simulink model "rc_second_order_open_close_loop_P_PI_PID_arduino"  (R2022b)
settings: Solver=FixedStepDiscrete  StartTime=0.0  StopTime=60.0  FixedStep=1e-3  RelTol=1e-3  EnableMultiTasking=on
undefined symbols (not defined in the file): DiscIntNeverNeededParam
libraries: arduinolib x10, simulink x1
settings Model: ExtModeTrigDuration=2  Creator=yasso  LastModifiedBy=yasso
settings OptimizationCC: EnhancedBackFolding=on  PassReuseOutputArgsAs=Individual arguments  ZeroExternalMemoryAtStartup=off  ZeroInternalMemoryAtStartup=off  MaxStackSize=64  OptimizeBlockOrder=speed  DifferentSizesBufferReuse=on  OptimizationCustomize=off  EfficientTunableParamExpr=on
settings DebuggingCC: ParameterTunabilityLossMsg=error
settings HardwareCC: ProdBitPerInt=16  ProdBitPerPointer=16  ProdBitPerSizeT=16  ProdBitPerPtrDiffT=16  ProdLargestAtomicFloat=None  ProdWordSize=8  ProdHWDeviceType=Atmel->AVR
settings SFSimCC: MATLABDynamicMemAlloc=off
settings RTWCC: Description=Embedded Coder  SystemTargetFile=ert.tlc  HardwareBoard=Arduino Uno  TLCOptions=-aInlineSetEventsForThisBaseRateFcn=TLC_FALSE -aSuppressMultiTaskScheduler=TLC_FALSE -aRateBasedStepFcn=1  TemplateMakefile=ert_default_tmf  Toolchain=Arduino AVR  BuildConfiguration=Faster Runs
settings CodeAppCC: ForceParamTrailComments=on  IgnoreCustomStorageClasses=off  OperatorAnnotations=on  SimulinkDataObjDesc=on  SFDataObjDesc=on  InsertBlockDesc=on
settings ERTTargetCC: SupportContinuousTime=on  SupportVariableSizeSignals=on  ExtModeTransport=3  ExtModeStaticAlloc=on  ExtModeAutomaticAllocSize=off  ExtModeStaticAllocSize=250  ExtModeMexFile=ext_xcp  ExtModeIntrfLevel=Level2 - Open

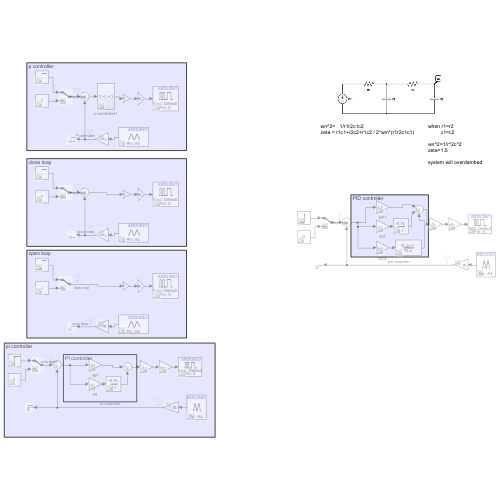
[thumbnail: Simulink's stored preview of the top-level diagram]
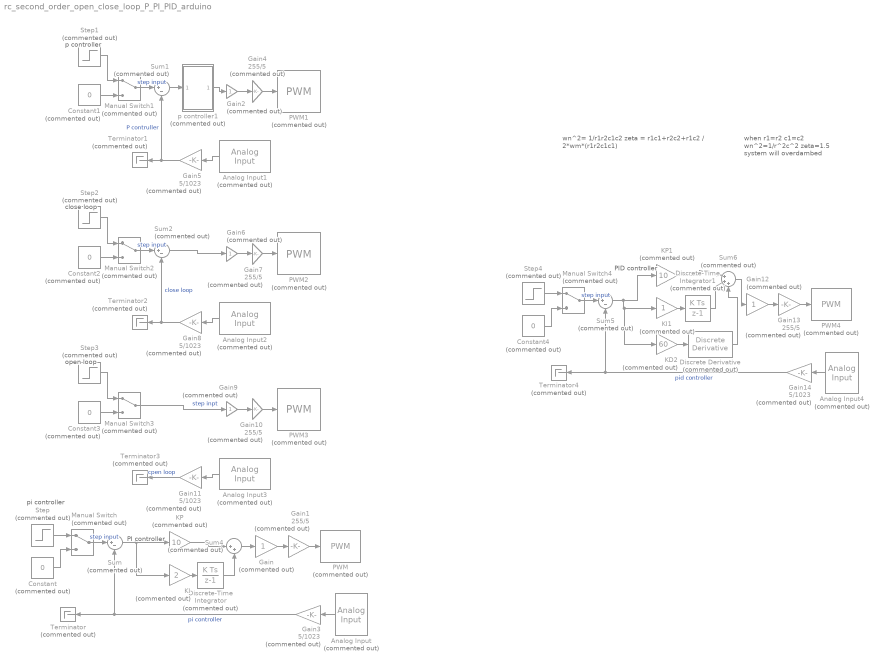
== system rc_second_order_open_close_loop_P_PI_PID_arduino ==
  note: pi controller
  note: PI controller
  note: p controller
  note: when r1=r2
      | c1=c2
      |
      | wn^2=1/r^2c^2
      | zeta=1.5
      |
      | system will overdambed
  note: wn^2= 1/r1r2c1c2
      | zeta = r1c1+r2c2+r1c2 / 2*wm*(r1r2c1c1)
  note: close loop
  note: open loop
  note: PID controller
  Analog Input{,1..4} (5 alike) : arduinolib/Analog Input  Commented=on  pinNumber=4  ReadResultsOnly=off  ConversionTriggerSource=Software  ExternalTriggerType=uint32( 0 )  OutputDataType=uint16  EnableConversionCompleteNotify=off  EnableOuputStatus=off  SampleTime=-1  blockPlatform=arduino
  Constant{,1..4} (5 alike) : Constant  Commented=on  Value=0
  Discrete Derivative : simulink/Discrete/Discrete Derivative  Commented=on  gainval=1.0  ICPrevScaledInput=0.0  OutMin=[]  OutMax=[]  OutDataType=fixdt(1, 16)  OutScaling=2^-10  DoSatur=off
  Discrete-Time Integrator : DiscreteIntegrator  Commented=on  SampleTime=-1  ICPrevOutput=DiscIntNeverNeededParam  ICPrevScaledInput=DiscIntNeverNeededParam
  Discrete-Time Integrator1 : DiscreteIntegrator  Commented=on  SampleTime=-1  ICPrevOutput=DiscIntNeverNeededParam  ICPrevScaledInput=DiscIntNeverNeededParam
  Gain{,2,6,9,12} (5 alike) : Gain  Commented=on
  Gain{1,4,7,10,13} (5 alike) : Gain  Commented=on  Gain=255/5
  Gain{3,5,8,11,14} (5 alike) : Gain  Commented=on  Gain=5/1023
  KD2 : Gain  Commented=on  Gain=60
  KI : Gain  Commented=on  Gain=2
  KI1 : Gain  Commented=on
  KP : Gain  Commented=on  Gain=10
  KP1 : Gain  Commented=on  Gain=10
  Manual Switch{,1..4} (5 alike) : ManualSwitch  Commented=on
  PWM{,1..4} (5 alike) : arduinolib/PWM  Commented=on  pinNumber=5  frequencyType=Default  desiredFrequency=490.2  achievableFrequency=490.2
  Step{,1..4} (5 alike) : Step  Commented=on  SampleTime=0
  Sum{,1..2,5} (4 alike) : Sum  Commented=on  Inputs=|+-
  Sum4 : Sum  Commented=on  Inputs=|++
  Sum6 : Sum  Commented=on  Inputs=|+++
  Terminator{,1..4} (5 alike) : Terminator  Commented=on
  p controller1 : Subsystem  Commented=on
  wires:
  Constant/1 -> Manual Switch/2
  Step/1 -> Manual Switch/1
  Gain/1 -> Gain1/1
  Gain1/1 -> PWM/1
  Analog Input/1 -> Gain3/1
  Gain3/1 -> Sum/2, Terminator/1  "pi controller"
  Manual Switch/1 -> Sum/1  "step input"
  Sum4/1 -> Gain/1
  p controller1/1(Out1) -> Gain2/1
  Sum1/1 -> p controller1/1(In1)
  Manual Switch1/1 -> Sum1/1  "step input"
  Gain5/1 -> Terminator1/1, Sum1/2  "P contruller"
  Analog Input1/1 -> Gain5/1
  Gain4/1 -> PWM1/1
  Gain2/1 -> Gain4/1
  Step1/1 -> Manual Switch1/1
  Constant1/1 -> Manual Switch1/2
  Constant2/1 -> Manual Switch2/2
  Step2/1 -> Manual Switch2/1
  Gain6/1 -> Gain7/1
  Gain7/1 -> PWM2/1
  Analog Input2/1 -> Gain8/1
  Gain8/1 -> Sum2/2, Terminator2/1  "close loop"
  Manual Switch2/1 -> Sum2/1  "step input"
  Sum2/1 -> Gain6/1
  Manual Switch3/1 -> Gain9/1  "step inpt"
  Gain11/1 -> Terminator3/1  "cpen loop"
  Analog Input3/1 -> Gain11/1
  Gain10/1 -> PWM3/1
  Gain9/1 -> Gain10/1
  Step3/1 -> Manual Switch3/1
  Constant3/1 -> Manual Switch3/2
  KP/1 -> Sum4/1
  Sum/1 -> KI/1, KP/1
  Discrete-Time Integrator/1 -> Sum4/2
  KI/1 -> Discrete-Time Integrator/1
  KI1/1 -> Discrete-Time Integrator1/1
  Discrete-Time Integrator1/1 -> Sum6/2
  Sum5/1 -> KP1/1, KD2/1, KI1/1
  KP1/1 -> Sum6/1
  Sum6/1 -> Gain12/1
  Manual Switch4/1 -> Sum5/1  "step input"
  Gain14/1 -> Terminator4/1, Sum5/2  "pid controller"
  Analog Input4/1 -> Gain14/1
  Gain13/1 -> PWM4/1
  Gain12/1 -> Gain13/1
  Step4/1 -> Manual Switch4/1
  Constant4/1 -> Manual Switch4/2
  KD2/1 -> Discrete Derivative/1
  Discrete Derivative/1 -> Sum6/3

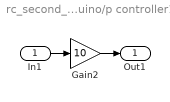
== system rc_second_order_open_close_loop_P_PI_PID_arduino/p controller1 ==
  In1 : Inport
  Gain2 : Gain  Gain=10
  Out1 : Outport
  wires:
  Gain2/1 -> Out1/1
  In1/1 -> Gain2/1
